simulink model "q4"  (R2026a)
settings: Solver=VariableStepAuto
settings Model: Creator=LAB_PC  LastModifiedBy=LAB_PC

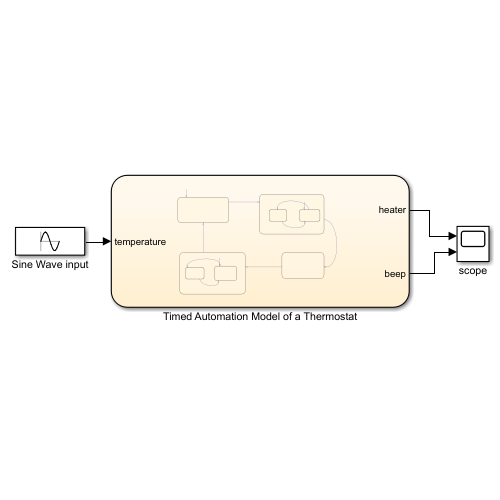
[thumbnail: Simulink's stored preview of the top-level diagram]
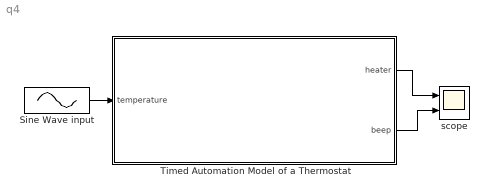
== system q4 ==
  Sine Wave input : Sin  Amplitude=5  Bias=24  SampleTime=0
  Timed Automation Model of a Thermostat : Stateflow chart  TreatAsAtomicUnit=on
  scope : Scope  NumInputPorts=2
      settings: ActiveDisplayYMinimum=-0.27097839560055903  ActiveDisplayYMaximum=1.2484044168994415
  wires:
  Sine Wave input/1 -> Timed Automation Model of a Thermostat/1(temperature)
  Timed Automation Model of a Thermostat/1(heater) -> scope/1
  Timed Automation Model of a Thermostat/2(beep) -> scope/2

== stateflow chart q4/Timed Automation Model of a Thermostat ==
  state Warn_Heating
    en: heater = 0;
    ex: beep = 0;
    state BeepOff
      en: beep = 0;
    state BeepOn
      en: beep = 1;
    Warn_Heating.BeepOn -> Warn_Heating.BeepOff : after(0.5, sec)
    (default) -> Warn_Heating.BeepOn
    Warn_Heating.BeepOff -> Warn_Heating.BeepOn : after(0.5,sec)
  state Cooling
    en:heater=0; beep=0;
  state Warn_Cooling
    en: heater = 1;
    ex: beep = 0;
    state BeepOn
      en: beep = 1;
    state BeepOff
      en: beep = 0;
    (default) -> Warn_Cooling.BeepOn
    Warn_Cooling.BeepOn -> Warn_Cooling.BeepOff : after(0.5, sec)
    Warn_Cooling.BeepOff -> Warn_Cooling.BeepOn : after(0.5,sec)
  state Heating
    en: heater = 1; beep = 0;
  (default) -> Cooling
  Cooling -> Warn_Heating : [temperature<22]
  Warn_Heating -> Heating : after(5,sec)
  Warn_Cooling -> Cooling : after(5,sec)
  Heating -> Warn_Cooling : [temperature>26]
  data: temperature input; heater output; beep output
